simulink model "d_DC_Motor"  (R2024b)
settings: Solver=VariableStepAuto  StartTime=0.0  StopTime=5  RelTol=1e-3
settings Model: Creator=Hp  LastModifiedBy=Hp

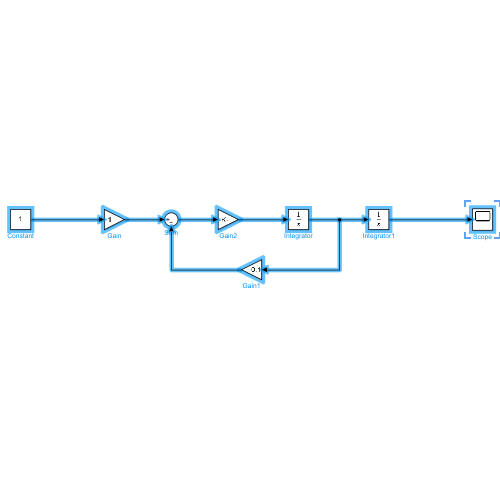
[thumbnail: Simulink's stored preview of the top-level diagram]
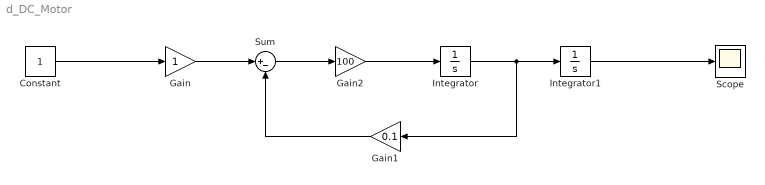
== system d_DC_Motor ==
  Constant : Constant
  Gain : Gain
  Gain1 : Gain  Gain=0.1
  Gain2 : Gain  Gain=100
  Integrator : Integrator
  Integrator1 : Integrator
  Scope : Scope
  Sum : Sum  Inputs=|+-
  wires:
  Constant/1 -> Gain/1
  Gain1/1 -> Sum/2
  Integrator/1 -> Gain1/1, Integrator1/1
  Gain/1 -> Sum/1
  Sum/1 -> Gain2/1
  Gain2/1 -> Integrator/1
  Integrator1/1 -> Scope/1
